simulink model "model_with_matlab_function"  (R2025b)
settings: Solver=ode45  StartTime=0.0  StopTime=10.0  RelTol=1e-3
PreLoadFcn:
  | callback_preload();
InitFcn:
  | callback_init();
StartFcn:
  | callback_start();
StopFcn:
  | callback_stop();
undefined symbols (not defined in the file or in its folder): amplitude_param, frequency_param, gain_param
libraries: simulink x1
CloseFcn:
  | callback_close();
settings Model: Creator=KoayXianCong  LastModifiedBy=KoayXianCong

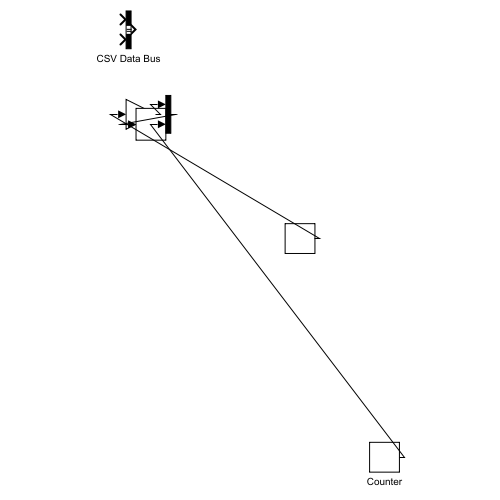
[thumbnail: Simulink's stored preview of the top-level diagram]
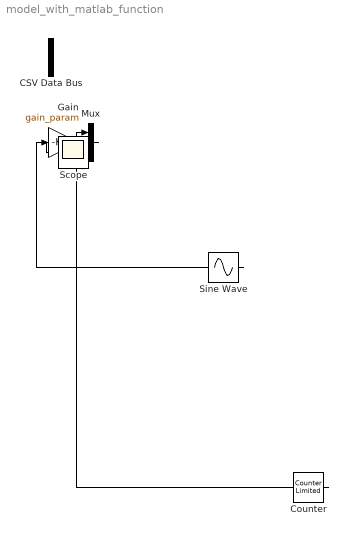
== system model_with_matlab_function ==
  CSV Data Bus : BusCreator  Inputs=2
  Counter : simulink/Sources/Counter Limited  uplimit=7  tsamp=-1
  Gain : Gain  Gain=gain_param
  Mux : Mux  Inputs=2
  Scope : Scope
  Sine Wave : Sin  Amplitude=amplitude_param  Frequency=frequency_param  SampleTime=0
  wires:
  Sine Wave/1 -> Gain/1
  Gain/1 -> Mux/1
  Counter/1 -> Mux/2
  Mux/1 -> Scope/1
